simulink model "simulation"  (R2015b)
settings: Solver=VariableStepAuto  StartTime=0.0  StopTime=1000  RelTol=1e-3
libraries: simulink x1
settings Model: Creator=timo  LastModifiedBy=timo

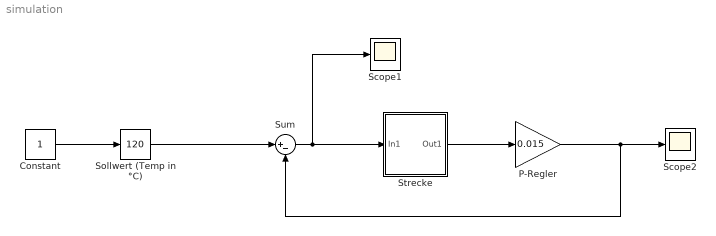
== system simulation ==
  Constant : Constant
  P-Regler : Gain  Gain=0.015
  Scope1 : Scope
  Scope2 : Scope
  Sollwert (Temp in °C) : simulink/Math Operations/Slider Gain  low=20  gain=120  high=120
  Strecke : Subsystem
  Sum : Sum  Inputs=|+-
  wires:
  Sum/1 -> Strecke/1(In1), Scope1/1
  Constant/1 -> Sollwert (Temp in °C)/1
  Sollwert (Temp in °C)/1 -> Sum/1
  P-Regler/1 -> Sum/2, Scope2/1
  Strecke/1(Out1) -> P-Regler/1

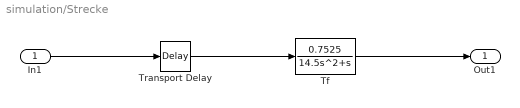
== system simulation/Strecke ==
  In1 : Inport
  Tf : TransferFcn  Numerator=[0.7525]  Denominator=[ 14.5 1 0]
  Transport Delay : TransportDelay  DelayTime=22.5
  Out1 : Outport
  wires:
  In1/1 -> Transport Delay/1
  Transport Delay/1 -> Tf/1
  Tf/1 -> Out1/1
